simulink library "LIB_TF_G_12_StepControl"  (Simulink 8.6)
settings: Solver=ode45  StartTime=0.0  StopTime=10.0  RelTol=1e-3
PreLoadFcn:
  | if exist('tl_preloadfcn','file'), tl_preloadfcn(gcs,402); end
PostLoadFcn:
  | if exist('tl_postloadfcn','file'), tl_postloadfcn(gcs,402); end
undefined symbols (not defined in the file or in its folder): ddv
libraries: tllib x2
(part 2 of 2)

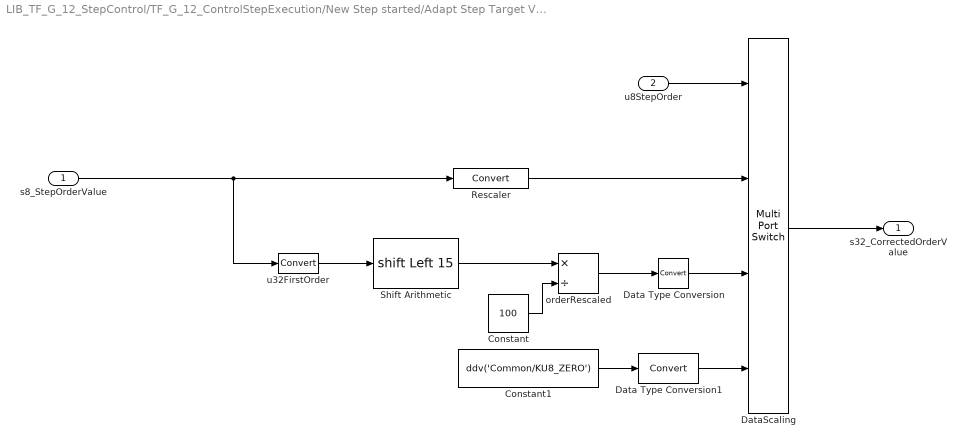
== system LIB_TF_G_12_StepControl/TF_G_12_ControlStepExecution/New Step started/Adapt Step Target Value ==
  s8_StepOrderValue : Inport
  u8StepOrder : Inport  Port=2
  Constant : Constant  Value=100  mask(TL_Constant){data={'date',738370.64164392359}}
      settings: CopyFcn=if exist('tl_reset_reviewflag') == 2, tl_reset_reviewflag(gcbh); end  DeleteFcn=if exist('delete_tlblock','file')==2,delete_tlblock(gcbh);end  NameChangeFcn=if exist('rename_tlblock','file')==2,rename_tlblock(gcbh);end  OpenFcn=if exist('tl_open_blockdlg','file')==2,tl_open_blockdlg(gcbh);else,open_system(gcbh,'parameter');end
      mask Help: eval(['if exist(''tl_online_help'',''file'') == 2, tl_online_help(''Topic'',''TL_Constant''),else, web([''jar:file:///'',matlabroot,''/help/toolbox/simulink/help.jar!/slref/' lower(get_param(gcbh,'Blocktype')) '.html''], ''-helpbrowser''),end'])
      mask Display: plot([-0.1, 1.05, NaN, -0.1, 1.05],[.01, .01, NaN, .99, .99]);
  Constant1 : Constant  Value=ddv('Common/KU8_ZERO')  mask(TL_Constant){data={'output',{'variable','Common/KU8_ZERO'},'date',738772.5296077315}}
      settings: CopyFcn=if exist('tl_reset_reviewflag') == 2, tl_reset_reviewflag(gcbh); end  DeleteFcn=if exist('delete_tlblock','file')==2,delete_tlblock(gcbh);end  NameChangeFcn=if exist('rename_tlblock','file')==2,rename_tlblock(gcbh);end  OpenFcn=if exist('tl_open_blockdlg','file')==2,tl_open_blockdlg(gcbh);else,open_system(gcbh,'parameter');end
      mask Help: eval(['if exist(''tl_online_help'',''file'') == 2, tl_online_help(''Topic'',''TL_Constant''),else, web([''jar:file:///'',matlabroot,''/help/toolbox/simulink/help.jar!/slref/' lower(get_param(gcbh,'Blocktype')) '.html''], ''-helpbrowser''),end'])
      mask Display: plot([-0.1, 1.05, NaN, -0.1, 1.05],[.01, .01, NaN, .99, .99]);
  Data Type Conversion : DataTypeConversion
  Data Type Conversion1 : DataTypeConversion
  DataScaling : MultiPortSwitch  DataPortOrder=Specify indices  Inputs=2  DataPortIndices={1,2}  DataPortForDefault=Additional data port  mask(TL_MultiPortSwitch){data={'output',{'type','Int32'},'date',738433.45357236115}}
      settings: CopyFcn=if exist('tl_reset_reviewflag') == 2, tl_reset_reviewflag(gcbh); end  DeleteFcn=if exist('delete_tlblock','file')==2,delete_tlblock(gcbh);end  NameChangeFcn=if exist('rename_tlblock','file')==2,rename_tlblock(gcbh);end  OpenFcn=if exist('tl_open_blockdlg','file')==2,tl_open_blockdlg(gcbh);else,open_system(gcbh,'parameter');end
      mask Help: eval(['if exist(''tl_online_help'',''file'') == 2, tl_online_help(''Topic'',''TL_MultiPortSwitch''),else, web([''jar:file:///'',matlabroot,''/help/toolbox/simulink/help.jar!/slref/' lower(get_param(gcbh,'Blocktype')) '.html''], ''-helpbrowser''),end'])
      mask Display: plot([-0.1, 1.05, NaN, -0.1, 1.05],[.01, .01, NaN, .99, .99]);
  Rescaler : DataTypeConversion  mask(TL_Rescaler){data={'output',{'type','Int32'},'date',738430.48060440971}}
      settings: DeleteFcn=if exist('delete_tlblock','file')==2,delete_tlblock(gcbh);end  NameChangeFcn=if exist('rename_tlblock','file')==2,rename_tlblock(gcbh);end  OpenFcn=if exist('tl_open_blockdlg','file')==2,tl_open_blockdlg(gcbh);else,open_system(gcbh,'parameter');end
      mask Help: eval(['if exist(''tl_online_help'',''file'') == 2, tl_online_help(''Topic'',''TL_Rescaler''),else, web([''jar:file:///'',matlabroot,''/help/toolbox/simulink/help.jar!/slref/' lower(get_param(gcbh,'Blocktype')) '.html''], ''-helpbrowser''),end'])
      mask Display: plot([-0.1, 1.05, NaN, -0.1, 1.05],[.01, .01, NaN, .99, .99]);
  Shift Arithmetic : ArithShift  LoadFcn=hBlOcK = gcbh; if strcmp(get_param(hBlOcK, 'LinkStatus'), 'resolved'), set_param(hBlOcK, 'LinkStatus', 'none'); set_param(hBlOcK, 'LoadFcn', ''); end; clear('hBlOcK');  BitShiftNumber=15  BitShiftDirection=Left  mask(TL_ArithShift){data={'logdata',{'loggingmode',1},'output',{'variable','SAD/Vars/Steps/u32OrderFullScale'},'date',738372.66674}}
      settings: DeleteFcn=if exist('delete_tlblock','file')==2,delete_tlblock(gcbh);end  NameChangeFcn=if exist('rename_tlblock','file')==2,rename_tlblock(gcbh);end  OpenFcn=if exist('tl_open_blockdlg','file')==2,tl_open_blockdlg(gcbh);else,open_system(gcbh,'parameter');end
      mask Help: eval(['if exist(''tl_online_help'',''file'') == 2, tl_online_help(''Topic'',''TL_ArithShift''),else, web([''jar:file:///'',matlabroot,''/help/toolbox/simulink/help.jar!/slref/' lower(get_param(gcbh,'Blocktype')) '.html''], ''-helpbrowser''),end'])
      mask Display: plot([-0.1, 1.05, NaN, -0.1, 1.05],[.01, .01, NaN, .99, .99]);
  orderRescaled : Product  Inputs=*/  RndMeth=Zero  mask(TL_Product){data={'logdata',{'loggingmode',1},'output',{'type','Int32'},'date',738370.71055672457}}
      settings: CopyFcn=if exist('tl_reset_reviewflag') == 2, tl_reset_reviewflag(gcbh); end  DeleteFcn=if exist('delete_tlblock','file')==2,delete_tlblock(gcbh);end  NameChangeFcn=if exist('rename_tlblock','file')==2,rename_tlblock(gcbh);end  OpenFcn=if exist('tl_open_blockdlg','file')==2,tl_open_blockdlg(gcbh);else,open_system(gcbh,'parameter');end
      mask Help: eval(['if exist(''tl_online_help'',''file'') == 2, tl_online_help(''Topic'',''TL_Product''),else, web([''jar:file:///'',matlabroot,''/help/toolbox/simulink/help.jar!/slref/' lower(get_param(gcbh,'Blocktype')) '.html''], ''-helpbrowser''),end'])
      mask Display: plot([-0.1, 1.05, NaN, -0.1, 1.05],[.01, .01, NaN, .99, .99]);
  u32FirstOrder : DataTypeConversion  mask(TL_Rescaler){data={'output',{'type','UInt32'},'date',738430.48040935188}}
      settings: DeleteFcn=if exist('delete_tlblock','file')==2,delete_tlblock(gcbh);end  NameChangeFcn=if exist('rename_tlblock','file')==2,rename_tlblock(gcbh);end  OpenFcn=if exist('tl_open_blockdlg','file')==2,tl_open_blockdlg(gcbh);else,open_system(gcbh,'parameter');end
      mask Help: eval(['if exist(''tl_online_help'',''file'') == 2, tl_online_help(''Topic'',''TL_Rescaler''),else, web([''jar:file:///'',matlabroot,''/help/toolbox/simulink/help.jar!/slref/' lower(get_param(gcbh,'Blocktype')) '.html''], ''-helpbrowser''),end'])
      mask Display: plot([-0.1, 1.05, NaN, -0.1, 1.05],[.01, .01, NaN, .99, .99]);
  s32_CorrectedOrderValue : Outport
  wires:
  Shift Arithmetic/1 -> orderRescaled/1
  Constant/1 -> orderRescaled/2
  u32FirstOrder/1 -> Shift Arithmetic/1
  orderRescaled/1 -> Data Type Conversion/1
  u8StepOrder/1 -> DataScaling/1
  DataScaling/1 -> s32_CorrectedOrderValue/1
  Data Type Conversion/1 -> DataScaling/3
  Rescaler/1 -> DataScaling/2
  s8_StepOrderValue/1 -> Rescaler/1, u32FirstOrder/1
  Constant1/1 -> Data Type Conversion1/1
  Data Type Conversion1/1 -> DataScaling/4

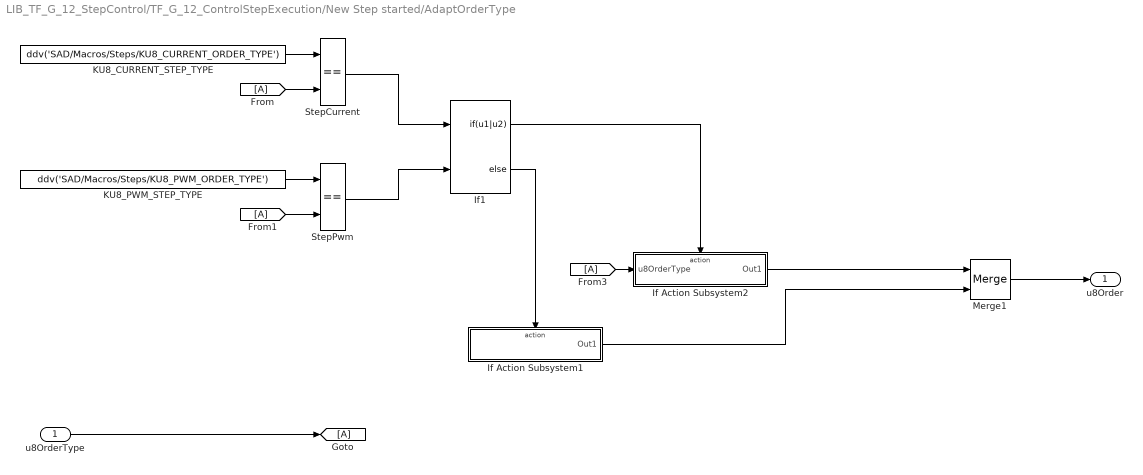
== system LIB_TF_G_12_StepControl/TF_G_12_ControlStepExecution/New Step started/AdaptOrderType ==
  u8OrderType : Inport  RequirementInfo={} %GIDa_d0932c2d_2946_4ca8_ae3e_f63aac2e144a
  If Action Subsystem1 : Subsystem  RequirementInfo={} %GIDa_efde54be_58e1_48f4_984b_1a55cd541708  TreatAsAtomicUnit=on
  If Action Subsystem2 : Subsystem  RequirementInfo={} %GIDa_7e05d702_bec6_4133_89e3_7df1c2d817b3  TreatAsAtomicUnit=on
  If1 : If  RequirementInfo={} %GIDa_230b83ff_c373_44fd_bf0d_fc368a5a2e7f  NumInputs=2  IfExpression=u1|u2
  KU8_CURRENT_STEP_TYPE : Constant  RequirementInfo={} %GIDa_98379601_80fc_49bf_9245_1ac9e089f011  Value=ddv('SAD/Macros/Steps/KU8_CURRENT_ORDER_TYPE')  OutDataTypeStr=uint8  mask(TL_Constant){data={'output',{'variable','SAD/Macros/Steps/KU8_CURRENT_ORDER_TYPE'},'date',738322.37700305553}}
      settings: CopyFcn=if exist('tl_reset_reviewflag','file')==2,tl_reset_reviewflag(gcbh);end  DeleteFcn=if exist('delete_tlblock','file')==2,delete_tlblock(gcbh);end  NameChangeFcn=if exist('rename_tlblock','file')==2,rename_tlblock(gcbh);end  OpenFcn=if exist('tl_open_blockdlg','file')==2,tl_open_blockdlg(gcbh);else,open_system(gcbh,'parameter');end
      mask Help: eval(['if exist(''tl_online_help'',''file'') == 2, tl_online_help(''Topic'',''TL_Constant''),else, web([''jar:file:///'',matlabroot,''/help/toolbox/simulink/help.jar!/slref/' lower(get_param(gcbh,'Blocktype')) '.html''], ''-helpbrowser''),end'])
      mask Display: plot([-0.05, 1.05, NaN, -0.05, 1.05],[.01, .01, NaN, .99, .99])
  KU8_PWM_STEP_TYPE : Constant  RequirementInfo={} %GIDa_29bcd219_c5cc_40dc_ab00_ad3704692ecd  Value=ddv('SAD/Macros/Steps/KU8_PWM_ORDER_TYPE')  OutDataTypeStr=uint8  mask(TL_Constant){data={'output',{'variable','SAD/Macros/Steps/KU8_PWM_ORDER_TYPE'},'date',738322.37718534726}}
      settings: CopyFcn=if exist('tl_reset_reviewflag','file')==2,tl_reset_reviewflag(gcbh);end  DeleteFcn=if exist('delete_tlblock','file')==2,delete_tlblock(gcbh);end  NameChangeFcn=if exist('rename_tlblock','file')==2,rename_tlblock(gcbh);end  OpenFcn=if exist('tl_open_blockdlg','file')==2,tl_open_blockdlg(gcbh);else,open_system(gcbh,'parameter');end
      mask Help: eval(['if exist(''tl_online_help'',''file'') == 2, tl_online_help(''Topic'',''TL_Constant''),else, web([''jar:file:///'',matlabroot,''/help/toolbox/simulink/help.jar!/slref/' lower(get_param(gcbh,'Blocktype')) '.html''], ''-helpbrowser''),end'])
      mask Display: plot([-0.05, 1.05, NaN, -0.05, 1.05],[.01, .01, NaN, .99, .99])
  Merge1 : Merge  RequirementInfo={} %GIDa_c83b2496_f2b0_4692_be7f_77f82a802315  InitialOutput=15  mask(TL_Merge){data={'output',{'name','u8NewRawOrderType'},'date',738370.3827106019}}
      settings: CopyFcn=if exist('tl_reset_reviewflag','file')==2,tl_reset_reviewflag(gcbh);end  DeleteFcn=if exist('delete_tlblock','file')==2,delete_tlblock(gcbh);end  NameChangeFcn=if exist('rename_tlblock','file')==2,rename_tlblock(gcbh);end  OpenFcn=if exist('tl_open_blockdlg','file')==2,tl_open_blockdlg(gcbh);else,open_system(gcbh,'parameter');end
      mask Help: eval(['if exist(''tl_online_help'',''file'') == 2, tl_online_help(''Topic'',''TL_Merge''),else, web([''jar:file:///'',matlabroot,''/help/toolbox/simulink/help.jar!/slref/' lower(get_param(gcbh,'Blocktype')) '.html''], ''-helpbrowser''),end'])
      mask Display: plot([-0.05, 1.05, NaN, -0.05, 1.05],[.01, .01, NaN, .99, .99])
  StepCurrent : RelationalOperator  RequirementInfo={} %GIDa_18ac9ebf_a7ed_4eb9_a4e9_7db870fd7569  Operator===  OutDataTypeStr=boolean  mask(TL_RelationalOperator){data={'logdata',{'loggingmode',1},'date',738367.48928825231}}
      settings: DeleteFcn=if exist('delete_tlblock','file')==2,delete_tlblock(gcbh);end  NameChangeFcn=if exist('rename_tlblock','file')==2,rename_tlblock(gcbh);end  OpenFcn=if exist('tl_open_blockdlg','file')==2,tl_open_blockdlg(gcbh);else,open_system(gcbh,'parameter');end
      mask Help: eval(['if exist(''tl_online_help'',''file'') == 2, tl_online_help(''Topic'',''TL_RelationalOperator''),else, web([''jar:file:///'',matlabroot,''/help/toolbox/simulink/help.jar!/slref/' lower(get_param(gcbh,'Blocktype')) '.html''], ''-helpbrowser''),end'])
      mask Display: plot([-0.05, 1.05, NaN, -0.05, 1.05],[.01, .01, NaN, .99, .99])
  StepPwm : RelationalOperator  RequirementInfo={} %GIDa_1f07f267_5fe9_402f_8d87_9ef376af47f7  Operator===  OutDataTypeStr=boolean  mask(TL_RelationalOperator){data={'logdata',{'loggingmode',1},'date',738367.48933934025}}
      settings: DeleteFcn=if exist('delete_tlblock','file')==2,delete_tlblock(gcbh);end  NameChangeFcn=if exist('rename_tlblock','file')==2,rename_tlblock(gcbh);end  OpenFcn=if exist('tl_open_blockdlg','file')==2,tl_open_blockdlg(gcbh);else,open_system(gcbh,'parameter');end
      mask Help: eval(['if exist(''tl_online_help'',''file'') == 2, tl_online_help(''Topic'',''TL_RelationalOperator''),else, web([''jar:file:///'',matlabroot,''/help/toolbox/simulink/help.jar!/slref/' lower(get_param(gcbh,'Blocktype')) '.html''], ''-helpbrowser''),end'])
      mask Display: plot([-0.05, 1.05, NaN, -0.05, 1.05],[.01, .01, NaN, .99, .99])
  u8Order : Outport  RequirementInfo={} %GIDa_7767866f_fef1_459c_9128_28c0971c6fc5
  wires:
  KU8_CURRENT_STEP_TYPE/1 -> StepCurrent/1
  StepCurrent/1 -> If1/1
  If1/2 -> If Action Subsystem1/Action
  KU8_PWM_STEP_TYPE/1 -> StepPwm/1
  StepPwm/1 -> If1/2
  If1/1 -> If Action Subsystem2/Action
  [A] -> StepCurrent/2
  [A] -> StepPwm/2
  [A] -> If Action Subsystem2/1(u8OrderType)
  u8OrderType/1 -> [A]
  Merge1/1 -> u8Order/1
  If Action Subsystem1/1(Out1) -> Merge1/2
  If Action Subsystem2/1(Out1) -> Merge1/1

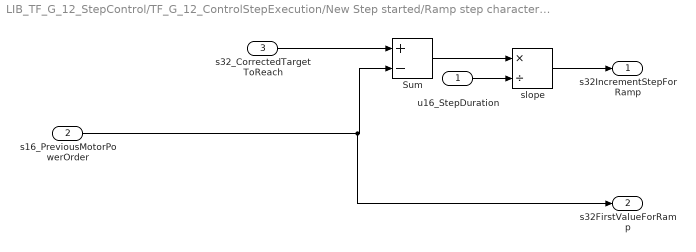
== system LIB_TF_G_12_StepControl/TF_G_12_ControlStepExecution/New Step started/Ramp step characteristics computation ==
  u16_StepDuration : Inport
  s16_PreviousMotorPowerOrder : Inport  Port=2
  s32_CorrectedTargetToReach : Inport  Port=3
  Sum : Sum  Inputs=+-  mask(TL_Sum){data={'logdata',{'loggingmode',1},'date',738370.70045474533}}
      settings: CopyFcn=if exist('tl_reset_reviewflag','file')==2,tl_reset_reviewflag(gcbh);end  DeleteFcn=if exist('delete_tlblock','file')==2,delete_tlblock(gcbh);end  NameChangeFcn=if exist('rename_tlblock','file')==2,rename_tlblock(gcbh);end  OpenFcn=if exist('tl_open_blockdlg','file')==2,tl_open_blockdlg(gcbh);else,open_system(gcbh,'parameter');end
      mask Help: eval(['if exist(''tl_online_help'',''file'') == 2, tl_online_help(''Topic'',''TL_Sum''),else, web([''jar:file:///'',matlabroot,''/help/toolbox/simulink/help.jar!/slref/' lower(get_param(gcbh,'Blocktype')) '.html''], ''-helpbrowser''),end'])
      mask Display: plot([-0.05, 1.05, NaN, -0.05, 1.05],[.01, .01, NaN, .99, .99])
  slope : Product  Inputs=*/  OutDataTypeStr=int32  RndMeth=Zero  mask(TL_Product){data={'logdata',{'loggingmode',1},'output',{'name','s16IncrementForRampStep'},'exceptionhandling',0,'date',738370.70063990739}}
      settings: CopyFcn=if exist('tl_reset_reviewflag','file')==2,tl_reset_reviewflag(gcbh);end  DeleteFcn=if exist('delete_tlblock','file')==2,delete_tlblock(gcbh);end  NameChangeFcn=if exist('rename_tlblock','file')==2,rename_tlblock(gcbh);end  OpenFcn=if exist('tl_open_blockdlg','file')==2,tl_open_blockdlg(gcbh);else,open_system(gcbh,'parameter');end
      mask Help: eval(['if exist(''tl_online_help'',''file'') == 2, tl_online_help(''Topic'',''TL_Product''),else, web([''jar:file:///'',matlabroot,''/help/toolbox/simulink/help.jar!/slref/' lower(get_param(gcbh,'Blocktype')) '.html''], ''-helpbrowser''),end'])
      mask Display: plot([-0.05, 1.05, NaN, -0.05, 1.05],[.01, .01, NaN, .99, .99])
  s32IncrementStepForRamp : Outport
  s32FirstValueForRamp : Outport  Port=2
  wires:
  s16_PreviousMotorPowerOrder/1 -> s32FirstValueForRamp/1, Sum/2
  s32_CorrectedTargetToReach/1 -> Sum/1
  Sum/1 -> slope/1
  slope/1 -> s32IncrementStepForRamp/1
  u16_StepDuration/1 -> slope/2

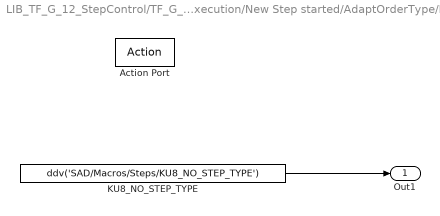
== system LIB_TF_G_12_StepControl/TF_G_12_ControlStepExecution/New Step started/AdaptOrderType/If Action Subsystem1 ==
  Action Port : ActionPort  RequirementInfo={} %GIDa_8c90ece7_90af_483e_9cad_cdc68c903bb6
  KU8_NO_STEP_TYPE : Constant  RequirementInfo={} %GIDa_88d5ae82_7c73_413a_a46d_5c66edb192c1  Value=ddv('SAD/Macros/Steps/KU8_NO_STEP_TYPE')  OutDataTypeStr=uint8  mask(TL_Constant){data={'output',{'variable','SAD/Macros/Steps/KU8_NO_STEP_TYPE'},'date',738322.44011927082}}
      settings: CopyFcn=if exist('tl_reset_reviewflag','file')==2,tl_reset_reviewflag(gcbh);end  DeleteFcn=if exist('delete_tlblock','file')==2,delete_tlblock(gcbh);end  NameChangeFcn=if exist('rename_tlblock','file')==2,rename_tlblock(gcbh);end  OpenFcn=if exist('tl_open_blockdlg','file')==2,tl_open_blockdlg(gcbh);else,open_system(gcbh,'parameter');end
      mask Help: eval(['if exist(''tl_online_help'',''file'') == 2, tl_online_help(''Topic'',''TL_Constant''),else, web([''jar:file:///'',matlabroot,''/help/toolbox/simulink/help.jar!/slref/' lower(get_param(gcbh,'Blocktype')) '.html''], ''-helpbrowser''),end'])
      mask Display: plot([-0.05, 1.05, NaN, -0.05, 1.05],[.01, .01, NaN, .99, .99])
  Out1 : Outport  RequirementInfo={} %GIDa_4ff01bec_1f37_45e3_ae87_576e41db2508
  wires:
  KU8_NO_STEP_TYPE/1 -> Out1/1

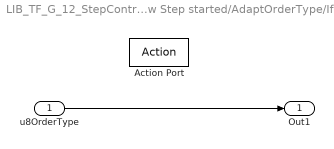
== system LIB_TF_G_12_StepControl/TF_G_12_ControlStepExecution/New Step started/AdaptOrderType/If Action Subsystem2 ==
  u8OrderType : Inport  RequirementInfo={} %GIDa_12107d9c_51c6_4b9c_ba46_1c9b53391efd
  Action Port : ActionPort  RequirementInfo={} %GIDa_1aa301e4_226a_435e_a06b_635fcf600117  ActionType=then
  Out1 : Outport  RequirementInfo={} %GIDa_f21eaf6f_27b3_4c29_92cc_8d5822c08ad3
  wires:
  u8OrderType/1 -> Out1/1
